simulink model "EconomicMPC_Simulink_Linear_mks_sep_5_cruise"  (R2022b)
settings: Solver=VariableStepAuto  StartTime=0.0  StopTime=4500  FixedStep=0.5  RelTol=1e-6
undefined symbols (not defined in the file): u0, x0
libraries: mpclib x1
settings Model: Creator=Mitarbeiter  LastModifiedBy=Mitarbeiter

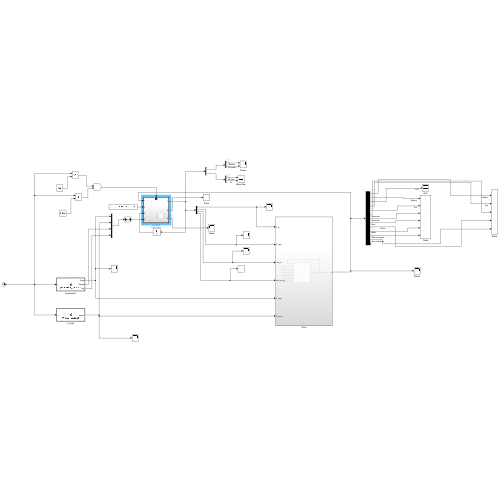
[thumbnail: Simulink's stored preview of the top-level diagram]
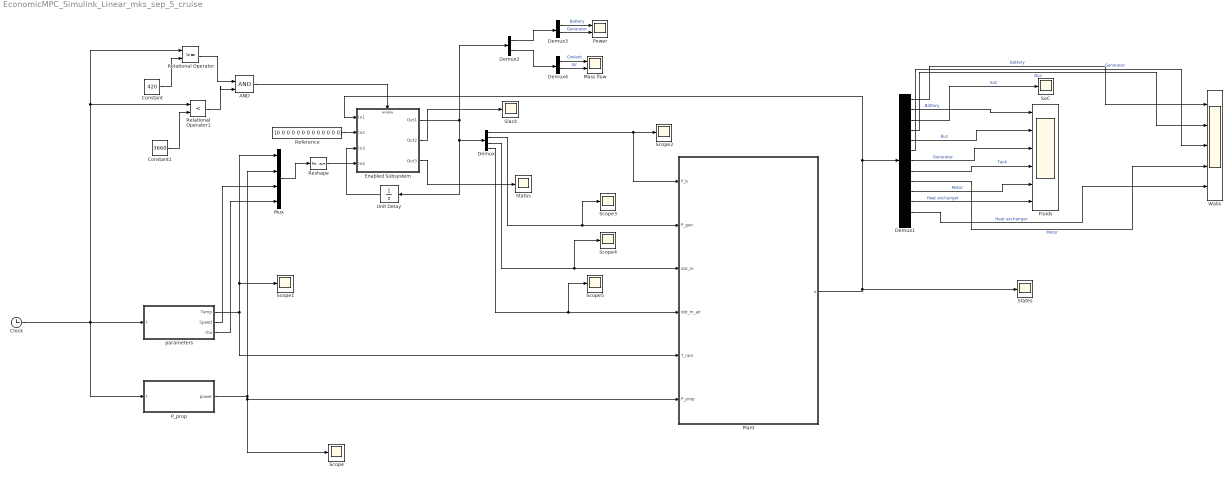
== system EconomicMPC_Simulink_Linear_mks_sep_5_cruise ==
  AND : Logic  IconShape=distinctive  AllPortsSameDT=off  OutDataTypeStr=boolean
  Clock : Clock
  Constant : Constant  Value=420
  Constant1 : Constant  Value=3660
  Demux : Demux
  Demux1 : Demux  Outputs=13
  Demux2 : Demux  Outputs=2
  Demux3 : Demux  Outputs=2
  Demux4 : Demux  Outputs=2
  Enabled Subsystem : Subsystem  TreatAsAtomicUnit=on
  Fluids : Scope  NumInputPorts=6
  Mass flow : Scope  NumInputPorts=2
  Mux : Mux
  P_prop : MATLAB Function  TreatAsAtomicUnit=on
  Plant : Subsystem
  Power : Scope  NumInputPorts=2
  Reference : Constant  Value=[0 0 0 0 0 0 0 0 0 0 0 0 0]  VectorParams1D=off
  Relational Operator : RelationalOperator  OutDataTypeStr=boolean  RndMeth=Simplest  InputSameDT=off
  Relational Operator1 : RelationalOperator  Operator=<  OutDataTypeStr=boolean  RndMeth=Simplest  InputSameDT=off
  Reshape : Reshape  OutputDimensionality=Row vector (2-D)
  Scope{,1..5} (6 alike) : Scope
  Slack : Scope
  SoC : Scope
  States : Scope
  Status : Scope
  Unit Delay : UnitDelay  InitialCondition=u0  SampleTime=-1  HasFrameUpgradeWarning=on
  Walls : Scope  NumInputPorts=5
  parameters : MATLAB Function  TreatAsAtomicUnit=on
  wires:
  Clock/1 -> Relational Operator1/1, Relational Operator/1, parameters/1(t), P_prop/1(t)
  parameters/1(Temp) -> Scope1/1, Mux/1, Plant/5(T_ram)
  P_prop/1(power) -> Scope/1, Plant/6(P_prop), Mux/2
  Plant/1(x) -> Enabled Subsystem/1(In1), Demux1/1, States/1
  Reference/1 -> Enabled Subsystem/2(In2)
  Demux/1 -> Scope2/1, Plant/1(P_b)
  Demux/2 -> Scope3/1, Plant/2(P_gen)
  Enabled Subsystem/1(Out1) -> Demux2/1, Demux/1, Unit Delay/1
  Mux/1 -> Reshape/1
  Unit Delay/1 -> Enabled Subsystem/3(In3)
  Reshape/1 -> Enabled Subsystem/4(In4)
  Demux1/3 -> SoC/1  "SoC"
  Enabled Subsystem/3(Out3) -> Status/1
  Demux/3 -> Scope4/1, Plant/3(dot_m)
  Demux/4 -> Scope5/1, Plant/4(dot_m_air)
  parameters/2(Speed) -> Mux/3
  Enabled Subsystem/2(Out2) -> Slack/1
  parameters/3(rho) -> Mux/4
  Demux4/1 -> Mass flow/1  "Coolant"
  Demux4/2 -> Mass flow/2  "Air"
  Demux3/2 -> Power/2  "Generator"
  Demux3/1 -> Power/1  "Battery"
  Demux2/1 -> Demux3/1
  Demux2/2 -> Demux4/1
  Demux1/1 -> Walls/1  "Battery"
  Demux1/2 -> Fluids/1  "Battery"
  Demux1/4 -> Walls/2  "Bus"
  Demux1/5 -> Fluids/2  "Bus"
  Demux1/6 -> Walls/3  "Generator"
  Demux1/7 -> Fluids/3  "Generator"
  Demux1/8 -> Fluids/4  "Tank"
  Demux1/9 -> Walls/4  "Motor"
  Demux1/10 -> Fluids/5  "Motor"
  Demux1/11 -> Fluids/6  "Heat exchanger"
  Demux1/12 -> Walls/5  "Heat exchanger"
  Constant/1 -> Relational Operator/2
  Constant1/1 -> Relational Operator1/2
  Relational Operator/1 -> AND/1
  Relational Operator1/1 -> AND/2
  AND/1 -> Enabled Subsystem/Enable

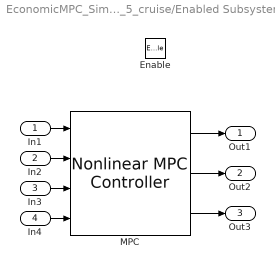
== system EconomicMPC_Simulink_Linear_mks_sep_5_cruise/Enabled Subsystem ==
  In1 : Inport
  In2 : Inport  Port=2
  In3 : Inport  Port=3
  In4 : Inport  Port=4
  Enable : EnablePort
  MPC : mpclib/Nonlinear MPC Controller  nlmpcobj=nlobj  UseObjectTs=on  UseMEX=off  md_enabled=on  mvtarget_enabled=off  param_enabled=off  cost_enabled=off  mvseq_enabled=off  stateseq_enabled=off  ovseq_enabled=off  slack_enabled=on  status_enabled=on  ov_min=off  ov_max=off  mv_min=off  mv_max=off  mvrate_min=off  mvrate_max=off  state_min=off  state_max=off  ov_weight=off  mv_weight=off  mvrate_weight=off  ecr_weight=off  nlp_initialize=off
  Out1 : Outport
  Out2 : Outport  Port=2
  Out3 : Outport  Port=3
  wires:
  In1/1 -> MPC/1
  In2/1 -> MPC/2
  In3/1 -> MPC/3
  In4/1 -> MPC/4
  MPC/1 -> Out1/1
  MPC/2 -> Out2/1
  MPC/3 -> Out3/1

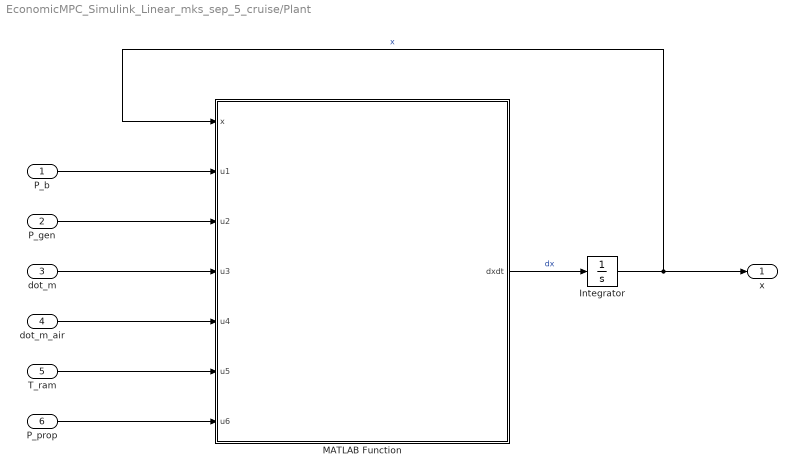
== system EconomicMPC_Simulink_Linear_mks_sep_5_cruise/Plant ==
  P_b : Inport
  P_gen : Inport  Port=2
  dot_m : Inport  Port=3
  dot_m_air : Inport  Port=4
  T_ram : Inport  Port=5
  P_prop : Inport  Port=6
  Integrator : Integrator  InitialCondition=x0
  MATLAB Function : MATLAB Function  TreatAsAtomicUnit=on
  x : Outport
  wires:
  MATLAB Function/1(dxdt) -> Integrator/1  "dx"
  Integrator/1 -> x/1, MATLAB Function/1(x)  "x"
  P_prop/1 -> MATLAB Function/7(u6)
  P_b/1 -> MATLAB Function/2(u1)
  dot_m/1 -> MATLAB Function/4(u3)
  dot_m_air/1 -> MATLAB Function/5(u4)
  T_ram/1 -> MATLAB Function/6(u5)
  P_gen/1 -> MATLAB Function/3(u2)

== matlab function EconomicMPC_Simulink_Linear_mks_sep_5_cruise/P_prop ==
  data: t input; power output
function power = P_prop_section2(t)
    % Section 2: Cruise (420 - 3660 s)
    power = 262e3 * ones(size(t)); % constant power
end

== matlab function EconomicMPC_Simulink_Linear_mks_sep_5_cruise/Plant/MATLAB Function ==
  data: x input; dxdt output; u1 input; u2 input; u3 input; u4 input; u5 input; u6 input
function dxdt = fcn(x,u1,u2,u3,u4,u5,u6)

 dxdt = aircraft_dynamics_linear_cruise(x,[u1;u2;u3;u4;u5;u6]);

== matlab function EconomicMPC_Simulink_Linear_mks_sep_5_cruise/parameters ==
  data: t input; Temp output; Speed output; rho output
function [Temp, Speed, rho] = parameters_section2(t)
    % ----- Section 2: Cruise -----
    t_cruise = 420;
    t_landing = 3660;

    % Altitude profile (constant at ~4000 ft)
    h = 4000 * ones(size(t));
    h = 0.3048 * h; % ft → m

    % Atmosphere
    Gamma = 1.4;
    R = 287.053;
    T_amp = -6.5e-3 * h + 15;
    a = sqrt(Gamma * R * (T_amp + 273.15));

    % Speed profile (constant at 125 knots)
    knot = 125 * ones(size(t));
    knot = 0.5144 * knot; % knots → m/s

    Mach = knot ./ a;
    Speed = Mach * 343;

    % Ram temperature
    Temp = T_amp .* (1+Mach.^2 * ((Gamma-1)/2));

    % Pressure altitude & density
    P0 = 101325;
    P = P0 * (1 - 2.25577e-5 * h).^5.25588;
    rho = P ./ (R * (T_amp+273.15));
end
